simulink model "Blocs"  (R2015a)
settings: Solver=ode45  StartTime=0.0  StopTime=1.0  RelTol=1e-3
libraries: dspsigops x1
settings Model: Creator=mlamraoui  LastModifiedBy=mlamraoui

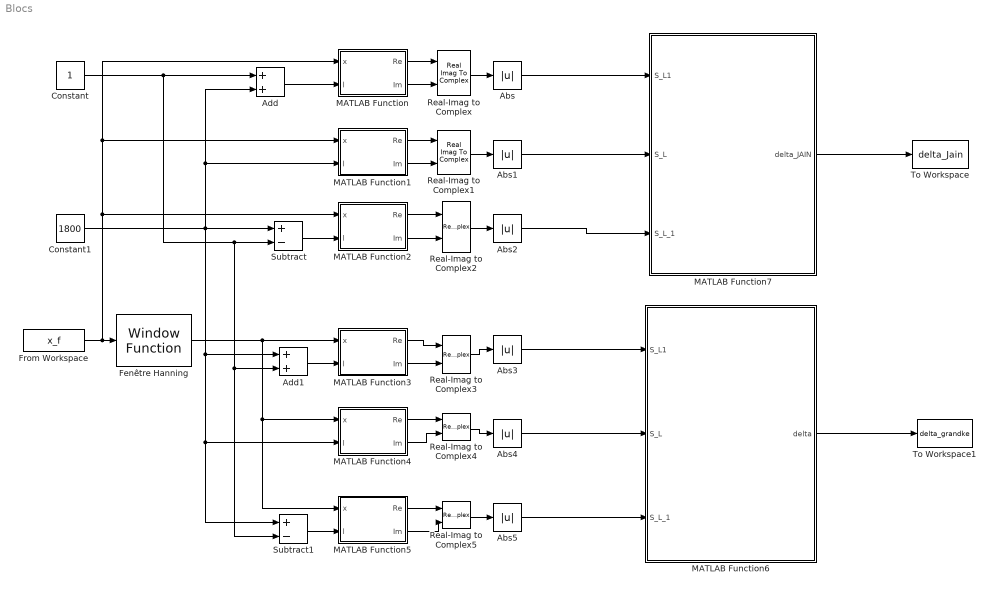
== system Blocs ==
  Abs{,1..5} (6 alike) : Abs
  Add : Sum
  Add1 : Sum
  Constant : Constant
  Constant1 : Constant  Value=1800
  "Fenêtre Hanning " : dspsigops/Window Function  winmode=Apply window to input  wintype=Hann  sampmode=Continuous  samptime=1  N=64  Rs=50  beta=10  winsamp=Symmetric  UserWindow=hamming  OptParams=off  UserParams={'symmetric'}  RowConvenienceOn=on  dataType=double  isSigned=on  wordLen=16  udDataType=sfix(16)  fracBitsMode=Best precision  numFracBits=15  roundingMode=Floor  overflowMode=off  numSidelobes=4  sidelobeLevel=-30
  From Workspace : FromWorkspace  VariableName=x_f
  MATLAB Function : MATLAB Function  TreatAsAtomicUnit=on
  MATLAB Function1 : MATLAB Function  TreatAsAtomicUnit=on
  MATLAB Function2 : MATLAB Function  TreatAsAtomicUnit=on
  MATLAB Function3 : MATLAB Function  TreatAsAtomicUnit=on
  MATLAB Function4 : MATLAB Function  TreatAsAtomicUnit=on
  MATLAB Function5 : MATLAB Function  TreatAsAtomicUnit=on
  MATLAB Function6 : MATLAB Function  TreatAsAtomicUnit=on
  MATLAB Function7 : MATLAB Function  TreatAsAtomicUnit=on
  Real-Imag to Complex{,1..5} (6 alike) : RealImagToComplex
  Subtract : Sum  Inputs=+-
  Subtract1 : Sum  Inputs=+-
  To Workspace : ToWorkspace  VariableName=delta_Jain  SaveFormat=Timeseries  SampleTime=-1
  To Workspace1 : ToWorkspace  VariableName=delta_grandke  SaveFormat=Timeseries  SampleTime=-1
  wires:
  From Workspace/1 -> MATLAB Function/1(x), MATLAB Function1/1(x), MATLAB Function2/1(x), "Fenêtre Hanning "/1
  "Fenêtre Hanning "/1 -> MATLAB Function5/1(x), MATLAB Function4/1(x), MATLAB Function3/1(x)
  Constant1/1 -> Add1/1, Subtract1/1, MATLAB Function4/2(l), Subtract/1, Add/2, MATLAB Function1/2(l)
  MATLAB Function/2(Im) -> Real-Imag to Complex/2
  MATLAB Function/1(Re) -> Real-Imag to Complex/1
  MATLAB Function1/1(Re) -> Real-Imag to Complex1/1
  MATLAB Function1/2(Im) -> Real-Imag to Complex1/2
  MATLAB Function2/1(Re) -> Real-Imag to Complex2/1
  MATLAB Function2/2(Im) -> Real-Imag to Complex2/2
  MATLAB Function3/1(Re) -> Real-Imag to Complex3/1
  MATLAB Function4/1(Re) -> Real-Imag to Complex4/1
  MATLAB Function4/2(Im) -> Real-Imag to Complex4/2
  MATLAB Function5/1(Re) -> Real-Imag to Complex5/1
  Real-Imag to Complex5/1 -> Abs5/1
  Real-Imag to Complex/1 -> Abs/1
  Real-Imag to Complex1/1 -> Abs1/1
  Real-Imag to Complex2/1 -> Abs2/1
  Real-Imag to Complex3/1 -> Abs3/1
  Real-Imag to Complex4/1 -> Abs4/1
  Add/1 -> MATLAB Function/2(l)
  Subtract/1 -> MATLAB Function2/2(l)
  Add1/1 -> MATLAB Function3/2(l)
  Constant/1 -> Subtract1/2, Add1/2, Subtract/2, Add/1
  Subtract1/1 -> MATLAB Function5/2(l)
  MATLAB Function5/2(Im) -> Real-Imag to Complex5/2
  MATLAB Function3/2(Im) -> Real-Imag to Complex3/2
  Abs4/1 -> MATLAB Function6/2(S_L)
  Abs3/1 -> MATLAB Function6/1(S_L1)
  Abs5/1 -> MATLAB Function6/3(S_L_1)
  Abs1/1 -> MATLAB Function7/2(S_L)
  Abs2/1 -> MATLAB Function7/3(S_L_1)
  Abs/1 -> MATLAB Function7/1(S_L1)
  MATLAB Function7/1(delta_JAIN) -> To Workspace/1
  MATLAB Function6/1(delta) -> To Workspace1/1

== matlab function Blocs/MATLAB Function1 ==
  data: x input; Re output; l input; Im output
function [Re,Im] = Goertzel(x,l)
 N= length(x);
 w = 2*pi*l/N;
 cw = cos(w); c = 2*cw;
 sw = sin(w);
 z1=0; z2=0; % initialisation
 for i = 1 : N
 z0 = x(i) + c*z1 - z2;
 z2 = z1;
 z1 = z0;
 end;
 Re= cw*z1 - z2;
 Im = sw*z1;

== matlab function Blocs/MATLAB Function ==
  data: x input; Re output; l input; Im output
function [Re,Im] = Goertzel(x,l)
 N= length(x);
 w = 2*pi*l/N;
 cw = cos(w); c = 2*cw;
 sw = sin(w);
 z1=0; z2=0; % initialisation
 for i = 1 : N
 z0 = x(i) + c*z1 - z2;
 z2 = z1;
 z1 = z0;
 end;
 Re= cw*z1 - z2;
 Im = sw*z1;

== matlab function Blocs/MATLAB Function2 ==
  data: x input; Re output; l input; Im output
function [Re,Im] = Goertzel(x,l)
 N= length(x);
 w = 2*pi*l/N;
 cw = cos(w); c = 2*cw;
 sw = sin(w);
 z1=0; z2=0; % initialisation
 for i = 1 : N
 z0 = x(i) + c*z1 - z2;
 z2 = z1;
 z1 = z0;
 end;
 Re= cw*z1 - z2;
 Im = sw*z1;

== matlab function Blocs/MATLAB Function3 ==
  data: x input; Re output; l input; Im output
function [Re,Im] = Goertzel(x,l)
 N= length(x);
 w = 2*pi*l/N;
 cw = cos(w); c = 2*cw;
 sw = sin(w);
 z1=0; z2=0; % initialisation
 for i = 1 : N
 z0 = x(i) + c*z1 - z2;
 z2 = z1;
 z1 = z0;
 end;
 Re= cw*z1 - z2;
 Im = sw*z1;

== matlab function Blocs/MATLAB Function4 ==
  data: x input; Re output; l input; Im output
function [Re,Im] = Goertzel(x,l)
 N= length(x);
 w = 2*pi*l/N;
 cw = cos(w); c = 2*cw;
 sw = sin(w);
 z1=0; z2=0; % initialisation
 for i = 1 : N
 z0 = x(i) + c*z1 - z2;
 z2 = z1;
 z1 = z0;
 end;
 Re= cw*z1 - z2;
 Im = sw*z1;

== matlab function Blocs/MATLAB Function5 ==
  data: x input; Re output; l input; Im output
function [Re,Im] = Goertzel(x,l)
 N= length(x);
 w = 2*pi*l/N;
 cw = cos(w); c = 2*cw;
 sw = sin(w);
 z1=0; z2=0; % initialisation
 for i = 1 : N
 z0 = x(i) + c*z1 - z2;
 z2 = z1;
 z1 = z0;
 end;
 Re= cw*z1 - z2;
 Im = sw*z1;

== matlab function Blocs/MATLAB Function6 ==
  data: S_L1 input; delta output; S_L input; S_L_1 input
function delta = GRANDKE(S_L1,S_L,S_L_1)
sig=sign(S_L1-S_L_1);
if(sig>0)
    alpha= S_L/S_L1;
    delta= sig*(2-alpha)/(1+alpha);
else 
    alpha= S_L/S_L_1;
    delta= sig*(2-alpha)/(1+alpha);
end
end

== matlab function Blocs/MATLAB Function7 ==
  data: S_L1 input; delta_JAIN output; S_L input; S_L_1 input
function delta_JAIN = JAIN(S_L1,S_L,S_L_1)
%#codegen

if (S_L1> S_L_1)%1er cas 0.5>delta>0 
    alpha=S_L1/S_L;
    delta_JAIN=alpha/(alpha+1);
else                 %2nd cas -0.5<delta<0 
    alpha=S_L_1/S_L;
    delta_JAIN=-alpha/(1+alpha);
end
end
